simulink model "pressureController"  (R2025b)
settings: Solver=FixedStepDiscrete  StartTime=0.0  StopTime=10.0  FixedStep=1/1000  RelTol=1e-3
undefined symbols (not defined in the file or in its folder): controller_mode, controller_modes, controllerGains
libraries: simulink x1, metux_library x1
settings Model: Creator=karadeli  LastModifiedBy=karadeli
settings OptimizationCC: DefaultParameterBehavior=Inlined  UseDivisionForNetSlopeComputation=on  GainParamInheritBuiltInType=on  UseFloatMulNetSlope=on  DefaultUnderspecifiedDataType=single  UseSpecifiedMinMax=on  InlineInvariantSignals=on  PassReuseOutputArgsAs=Individual arguments  ZeroExternalMemoryAtStartup=off  ZeroInternalMemoryAtStartup=off  NoFixptDivByZeroProtection=on  EfficientFloat2IntCast=on  LifeSpan=1  OptimizeBlockOrder=speed  DifferentSizesBufferReuse=on  EfficientTunableParamExpr=on
settings DebuggingCC: ParamSuppressDoubleToSinglePrecisionLossMsg=on  ParameterTunabilityLossMsg=error
settings HardwareCC: ProdBitPerPointer=32.0  ProdBitPerSizeT=32.0  ProdBitPerPtrDiffT=32.0  ProdLargestAtomicInteger=Long  ProdLargestAtomicFloat=Double  ProdWordSize=32.0  ProdLongLongMode=on  ProdHWDeviceType=ARM Compatible->ARM Cortex-M
settings SFSimCC: MATLABDynamicMemAlloc=off
settings RTWCC: SystemTargetFile=ert.tlc  GenCodeOnly=on  TemplateMakefile=ert_default_tmf  BuildConfiguration=Faster Runs  TargetLang=C++  Description=Embedded Coder
settings CodeAppCC: ForceParamTrailComments=on  IgnoreCustomStorageClasses=off  OperatorAnnotations=on  SimulinkDataObjDesc=on  SFDataObjDesc=on  CustomSymbolStrGlobalVar=rt$N$M  CustomSymbolStrType=$N$M  CustomSymbolStrFcn=$N$M$F  CustomSymbolStrMacro=$N$M  InsertBlockDesc=on
settings ERTTargetCC: RootIOFormat=Structure reference  ERTCustomFileTemplate=example_file_process.tlc  ERTFilePackagingFormat=CompactWithDataFile  TargetLangStandard=C++11 (ISO)  GenerateSampleERTMain=on  IncludeMdlTerminateFcn=off  CombineSignalStateStructs=on  SuppressErrorStatus=on  SupportAbsoluteTime=off  CodeInterfacePackaging=C++ class  SubcomponentCodeInterfacePackaging=C++ class  SupportComplex=off  SupportNonInlinedSFcns=on

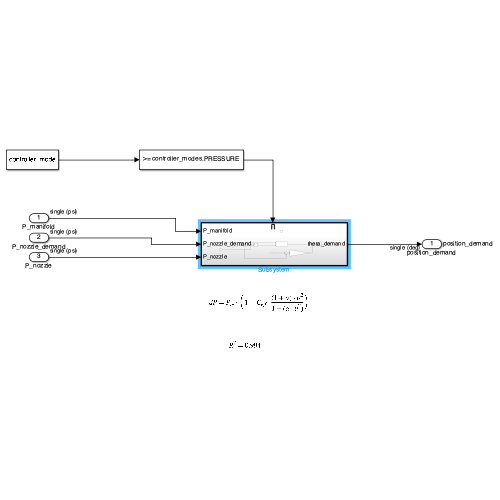
[thumbnail: Simulink's stored preview of the top-level diagram]
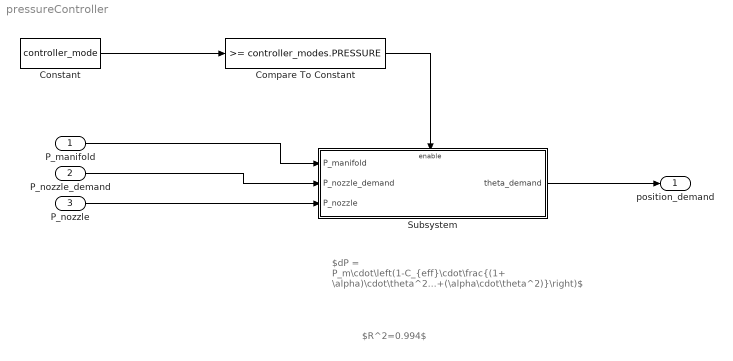
== system pressureController ==
  note: $R^2=0.994$
  note: $dP = P_m\cdot\left(1-C_{eff}\cdot\frac{(1+ \alpha)\cdot\theta^2}{1+(\alpha\cdot\theta^2)}\right)$
  P_manifold : Inport  OutDataTypeStr=single  Unit=psi  PortDimensions=1
  P_nozzle_demand : Inport  Port=2  OutDataTypeStr=single  Unit=psi  PortDimensions=1
  P_nozzle : Inport  Port=3  OutDataTypeStr=single  Unit=psi  PortDimensions=1
  Compare To Constant : simulink/Logic and Bit Operations/Compare To Constant  relop=>=  const=controller_modes.PRESSURE  OutDataTypeStr=boolean
  Constant : Constant  Value=controller_mode  SampleTime=-1
  Subsystem : Subsystem
  position_demand : Outport  SignalName=position_demand  OutDataTypeStr=single  Unit=deg
  wires:
  P_manifold/1 -> Subsystem/1(P_manifold)
  P_nozzle_demand/1 -> Subsystem/2(P_nozzle_demand)
  Subsystem/1(theta_demand) -> position_demand/1
  Constant/1 -> Compare To Constant/1
  Compare To Constant/1 -> Subsystem/Enable
  P_nozzle/1 -> Subsystem/3(P_nozzle)

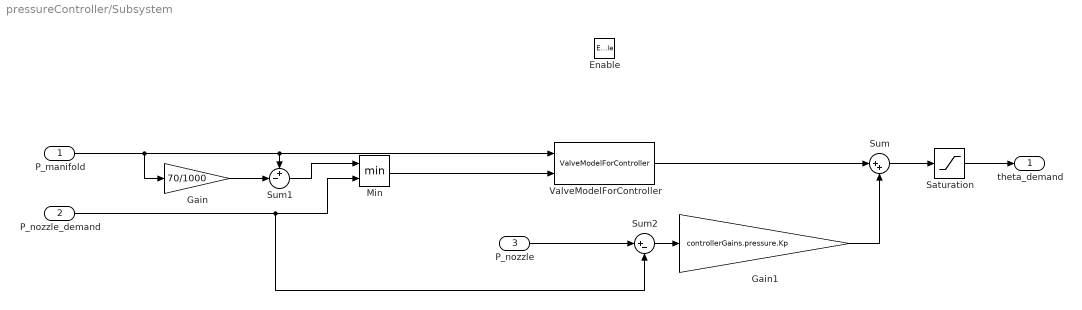
== system pressureController/Subsystem ==
  P_manifold : Inport
  P_nozzle_demand : Inport  Port=2
  P_nozzle : Inport  Port=3
  Enable : EnablePort  StatesWhenEnabling=reset
  Gain : Gain  Gain=70/1000
  Gain1 : Gain  Gain=controllerGains.pressure.Kp
  Min : MinMax  Inputs=2
  Saturation : Saturate  UpperLimit=1080  LowerLimit=0
  Sum : Sum  Inputs=|++
  Sum1 : Sum  Inputs=+-|
  Sum2 : Sum  Inputs=|+-
  ValveModelForController : metux_library/ValveModelForController  alpha=51.8534  C_max=0.9197
  theta_demand : Outport  OutputWhenDisabled=reset  InitialOutput=0
  wires:
  ValveModelForController/1 -> Sum/1
  Saturation/1 -> theta_demand/1
  Sum1/1 -> Min/1
  Gain/1 -> Sum1/2
  P_manifold/1 -> Sum1/1, ValveModelForController/1, Gain/1
  P_nozzle_demand/1 -> Sum2/2, Min/2
  Min/1 -> ValveModelForController/2
  P_nozzle/1 -> Sum2/1
  Gain1/1 -> Sum/2
  Sum/1 -> Saturation/1
  Sum2/1 -> Gain1/1
